simulink library "INT_Tra_Grip"  (R2016b)
settings: Solver=VariableStepAuto  StartTime=0.0  StopTime=10.0  RelTol=1e-3
settings Model: Creator=Administrator  LastModifiedBy=Administrator

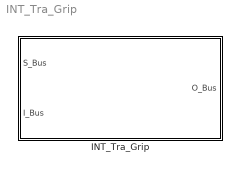
== system INT_Tra_Grip ==
  INT_Tra_Grip : Subsystem

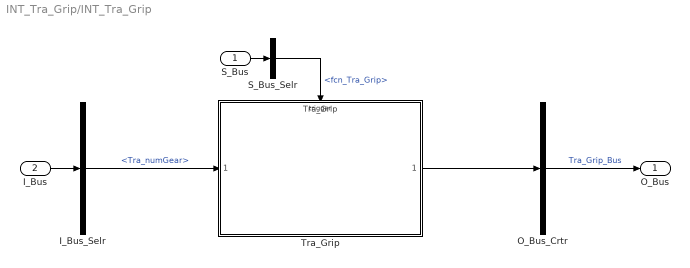
== system INT_Tra_Grip/INT_Tra_Grip ==
  S_Bus : Inport
  I_Bus : Inport  Port=2
  I_Bus_Selr : BusSelector  OutputSignals=Tra_numGear
  O_Bus_Crtr : BusCreator  Inputs=1
  S_Bus_Selr : BusSelector  OutputSignals=fcn_Tra_Grip
  Tra_Grip : ModelReference  ModelNameDialog=Tra_Grip  SimulationMode=Normal  ModelReferenceVersion=1.5  TriggerPortName=function  TriggerPortTriggerType=function-call  TriggerPortStatesWhenEnabling=held
  O_Bus : Outport
  wires:
  S_Bus_Selr/1 -> Tra_Grip/Trigger  "<fcn_Tra_Grip>"
  S_Bus/1 -> S_Bus_Selr/1
  I_Bus/1 -> I_Bus_Selr/1
  I_Bus_Selr/1 -> Tra_Grip/1  "<Tra_numGear>"
  O_Bus_Crtr/1 -> O_Bus/1  "Tra_Grip_Bus"
  Tra_Grip/1 -> O_Bus_Crtr/1
